simulink model "VG_C_code"  (R2024b)
settings: Solver=VariableStepAuto  StartTime=0.0  StopTime=10.0  RelTol=1e-3
settings Model: Creator=luigi  LastModifiedBy=luigi
settings SFSimCC: SimCustomHeaderCode="#include \"SVPWM_Full_singlePrecision.h\""  SimUserSources=SVPWM_Full_singlePrecision.c  SimDebugExecutionForCustomCode=on  DefaultCustomCodeDeterministicFunctions=All

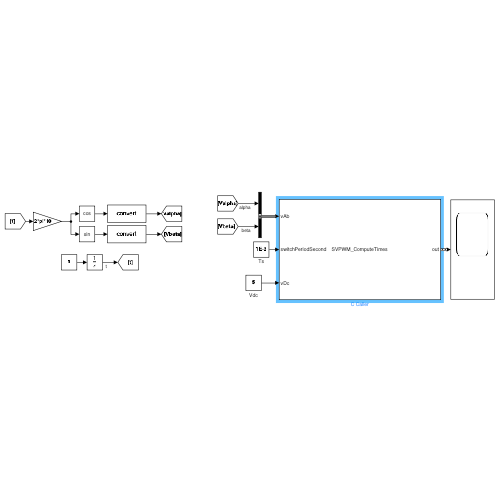
[thumbnail: Simulink's stored preview of the top-level diagram]
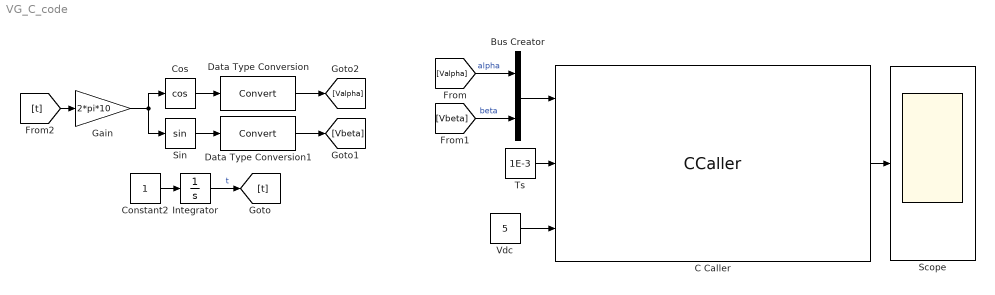
== system VG_C_code ==
  Bus Creator : BusCreator  Inputs=2
  C Caller : CCaller  FunctionName=SVPWM_ComputeTimes  PortSpecificationStruct="%)30     .    0 <   8    (     @         %    \"     0    !     0         %  0 \"0    $    _    07)G3F%M90  4&]R=$YA;64 4V-O<&4     26YD97@     5'EP90      4VEZ90      27-';&]B86P   X    P    !@    @    $          4    (     0    ,    !         !   P!O=70 #@   #     &    \"     0         !0    @    !     P    $         $  # &]U=  .    .     8    (    !          %    \"     $    &     0         0   ...(+2116 chars)"
  Constant2 : Constant
  Cos : Trigonometry  Operator=cos
  Data Type Conversion : DataTypeConversion  SaturateOnIntegerOverflow=off  RndMeth=Floor
  Data Type Conversion1 : DataTypeConversion  SaturateOnIntegerOverflow=off  RndMeth=Floor
  Gain : Gain  Gain=2*pi*10
  Integrator : Integrator
  Scope : Scope
  Sin : Trigonometry
  Ts : Constant  Value=1E-3  OutDataTypeStr=single
  Vdc : Constant  Value=5  OutDataTypeStr=single
  wires:
  Gain/1 -> Cos/1, Sin/1
  Sin/1 -> Data Type Conversion1/1
  Constant2/1 -> Integrator/1
  Integrator/1 -> [t]  "t"
  [t] -> Gain/1
  Cos/1 -> Data Type Conversion/1
  [Valpha] -> Bus Creator/1  "alpha"
  Ts/1 -> C Caller/2
  Vdc/1 -> C Caller/3
  Data Type Conversion/1 -> [Valpha]
  Data Type Conversion1/1 -> [Vbeta]
  C Caller/1 -> Scope/1
  Bus Creator/1 -> C Caller/1
  [Vbeta] -> Bus Creator/2  "beta"
